simulink model "R7014E_DoubleTankSim2018b_works_on_A"  (R2018a)
settings: Solver=ode5  StartTime=0.0  StopTime=500  FixedStep=0.02  RelTol=1e-3  EnableMultiTasking=on
values from neighbouring files (symbols this model uses):
  A = [a_1*(-1/sqrt(2*g*(h1+EqPoint))) 0 ... (first row only)    [myTank.m]
  B = [6.95/36.2; 0]    [myTank.m]
  C = [0 1]    [myTank.m]
  EqPoint = h_2.signals.values(end)    [myTank.m]
  K = (P*C' + N*0)/[0 1]    [myTank.m]
Description:
  | Double tank process simulation model
  | V1.0
  | 
  | Author: Wolfgang Birk, LTU
settings Model: MinMaxOverflowLogging=ForceOff  Creator=wolfgang  LastModifiedBy=oskwij-4
settings DataIOCC: LimitDataPoints=on  SaveFormat=Array  SignalLoggingSaveFormat=ModelDataLogs
settings OptimizationCC: ExpressionDepthLimit=2147483647  LifeSpan=inf
settings DebuggingCC: UnderspecifiedInitializationDetection=Classic  MergeDetectMultiDrivingBlocksExec=none  SolverPrmCheckMsg=warning  FcnCallInpInsideContextMsg=warning  StateNameClashWarn=warning  SFUnexpectedBacktrackingDiag=warning  SFNoUnconditionalDefaultTransitionDiag=warning  SFExecutionAtInitializationDiag=none
settings HardwareCC: ProdBitPerPointer=32  ProdBitPerSizeT=32  ProdBitPerPtrDiffT=32  ProdLargestAtomicFloat=None  ProdIntDivRoundTo=Undefined  ProdEndianess=Unspecified  ProdWordSize=32  ProdHWDeviceType=32-bit Generic
settings ModelReferenceCC: PropagateSignalLabelsOutOfModel=off
settings CodeAppCC: StateflowObjectComments=on
settings GRTTargetCC: TargetLangStandard=C89/C90 (ANSI)  GeneratePreprocessorConditionals=Disable all
settings ConfigComp: CovMetricSettings=dw  CovHtmlReporting=on  CovSaveCumulativeToWorkspaceVar=on  CovSaveSingleToWorkspaceVar=on  CovExternalEMLEnable=off

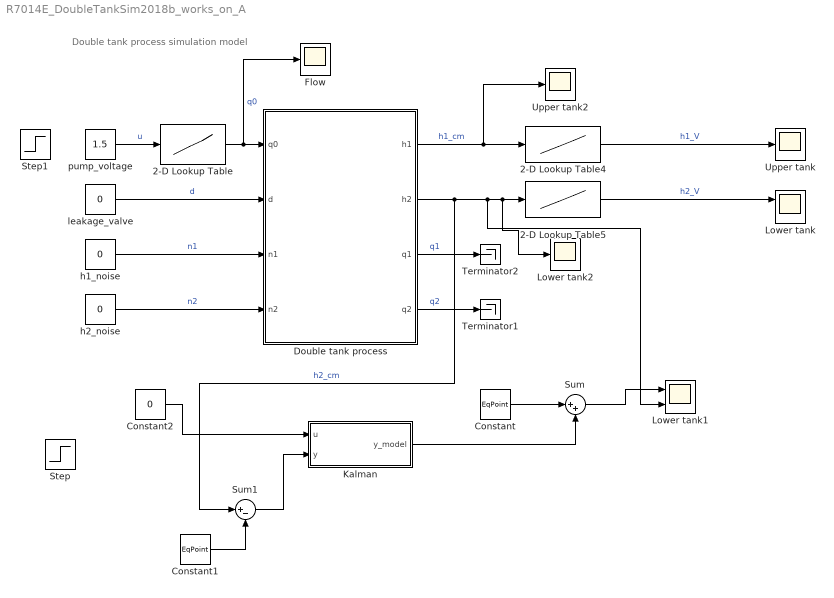
== system R7014E_DoubleTankSim2018b_works_on_A ==
  note: Double tank process simulation model
  2-D Lookup Table : Lookup_n-D  NumberOfTableDimensions=1  BreakpointsForDimension1=x  BreakpointsForDimension2=[1:3]  Table=y  RndMeth=Simplest  InputSameDT=on  mask{x=[0,1,2,3,4,5,6,7,8,9,10], y=[0, 22.23, 28.39, 33.5, 37.5, 41.0, 43.18, 46.9, 48.58, 50.37, 52.97]}
      mask prompts: x "Values on x-axis"; y "Values on y-axis"
  2-D Lookup Table4 : Lookup_n-D  NumberOfTableDimensions=1  BreakpointsForDimension1=x  BreakpointsForDimension2=[1:3]  Table=y  RndMeth=Simplest  InputSameDT=on  mask{x=[0, 2.9, 5.3, 6.5, 8.0, 9.0, 10.1, 11.1, 12.3, 14.0, 15.1], y=[0, 0.47, 2.27, 3.2, 4.3, 5.2, 6.1, 6.8, 7.75, 8.9, 9.8]}
      mask prompts: x "Values on x-axis"; y "Values on y-axis"
  2-D Lookup Table5 : Lookup_n-D  NumberOfTableDimensions=1  BreakpointsForDimension1=x  BreakpointsForDimension2=[1:3]  Table=y  RndMeth=Simplest  InputSameDT=on  mask{x=[0, 3.0, 5.4, 6.9, 7.6, 8.5, 9.5, 10.5, 12.1, 13.6, 14.6], y=[0, 0.83, 2.68, 3.9, 4.5, 5.2, 6.0, 6.9, 8.4, 9.4, 10.0]}
      mask prompts: x "Values on x-axis"; y "Values on y-axis"
  Constant : Constant  Value=EqPoint
  Constant1 : Constant  Value=EqPoint
  Constant2 : Constant  Value=0
  Double tank process : Subsystem  mask{At=33, Ao=0.17, hmax=15.5}
      mask prompts: At "Tank area (cm^2)"; Ao "Opening area (cm^2)"; hmax "Tank height (cm)"
      mask help: Double tank process parameters
  Flow : Scope
  Kalman : Subsystem
  Lower tank : Scope  NumInputPorts=2
  Lower tank1 : Scope  NumInputPorts=2
  "Lower tank2 " : Scope
  Step : Step  Time=250  After=0.1  SampleTime=0
  Step1 : Step  Time=250  Before=2  After=2.1  SampleTime=0
  Sum : Sum  Inputs=|++
  Sum1 : Sum  Inputs=|+-
  Terminator1 : Terminator
  Terminator2 : Terminator
  Upper tank : Scope
  Upper tank2 : Scope
  h1_noise : Constant  Value=0
  h2_noise : Constant  Value=0
  leakage_valve : Constant  Value=0
  pump_voltage : Constant  Value=1.5
  wires:
  2-D Lookup Table4/1 -> Upper tank/1  "h1_V"
  leakage_valve/1 -> Double tank process/2(d)  "d"
  2-D Lookup Table/1 -> Flow/1, Double tank process/1(q0)  "q0"
  Double tank process/1(h1) -> Upper tank2/1, 2-D Lookup Table4/1  "h1_cm"
  Double tank process/2(h2) -> Sum1/1, Lower tank1/2, "Lower tank2 "/1, 2-D Lookup Table5/1  "h2_cm"
  Double tank process/4(q2) -> Terminator1/1  "q2"
  2-D Lookup Table5/1 -> Lower tank/1  "h2_V"
  Double tank process/3(q1) -> Terminator2/1  "q1"
  h1_noise/1 -> Double tank process/3(n1)  "n1"
  h2_noise/1 -> Double tank process/4(n2)  "n2"
  Kalman/1("y_model ") -> Sum/2
  Constant/1 -> Sum/1
  Sum/1 -> Lower tank1/1
  Constant1/1 -> Sum1/2
  Sum1/1 -> Kalman/2(y)
  Constant2/1 -> Kalman/1(u)
  pump_voltage/1 -> 2-D Lookup Table/1  "u"

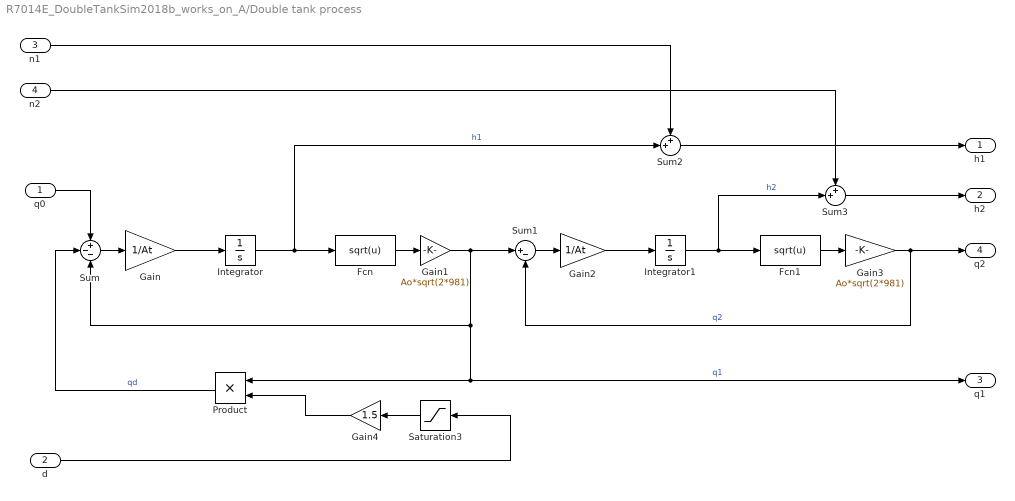
== system R7014E_DoubleTankSim2018b_works_on_A/Double tank process ==
  q0 : Inport
  d : Inport  Port=2
  n1 : Inport  Port=3
  n2 : Inport  Port=4
  Fcn : Fcn  Expr=sqrt(u)
  Fcn1 : Fcn  Expr=sqrt(u)
  Gain : Gain  Gain=1/At
  Gain1 : Gain  Gain=Ao*sqrt(2*981)
  Gain2 : Gain  Gain=1/At
  Gain3 : Gain  Gain=Ao*sqrt(2*981)
  Gain4 : Gain  Gain=1.5
  Integrator : Integrator  InitialCondition=EqPoint  LimitOutput=on  UpperSaturationLimit=hmax  LowerSaturationLimit=0
  Integrator1 : Integrator  InitialCondition=EqPoint  LimitOutput=on  UpperSaturationLimit=hmax  LowerSaturationLimit=0
  Product : Product  RndMeth=Zero
  Saturation3 : Saturate  UpperLimit=1  LowerLimit=0
  Sum : Sum  Inputs=+--
  Sum1 : Sum  Inputs=|+-
  Sum2 : Sum  Inputs=++|
  Sum3 : Sum  Inputs=++|
  h1 : Outport
  h2 : Outport  Port=2
  q1 : Outport  Port=3
  q2 : Outport  Port=4
  wires:
  Sum/1 -> Gain/1
  Gain/1 -> Integrator/1
  Fcn/1 -> Gain1/1
  Gain1/1 -> Sum1/1, Product/1, q1/1, Sum/3  "q1"
  Sum1/1 -> Gain2/1
  Gain2/1 -> Integrator1/1
  Fcn1/1 -> Gain3/1
  Gain3/1 -> Sum1/2, q2/1  "q2"
  q0/1 -> Sum/1
  Integrator/1 -> Sum2/2, Fcn/1  "h1"
  Product/1 -> Sum/2  "qd"
  d/1 -> Saturation3/1
  Integrator1/1 -> Sum3/2, Fcn1/1  "h2"
  Saturation3/1 -> Gain4/1
  Gain4/1 -> Product/2
  Sum2/1 -> h1/1
  n1/1 -> Sum2/1
  Sum3/1 -> h2/1
  n2/1 -> Sum3/1

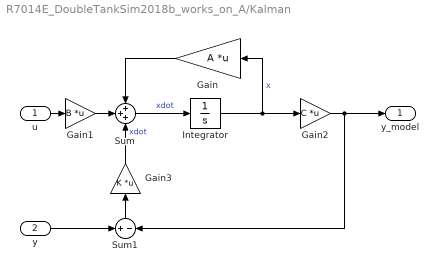
== system R7014E_DoubleTankSim2018b_works_on_A/Kalman ==
  u : Inport
  y : Inport  Port=2
  Gain : Gain  Gain=A  Multiplication=Matrix(K*u)
  Gain1 : Gain  Gain=B  Multiplication=Matrix(K*u)
  Gain2 : Gain  Gain=C  Multiplication=Matrix(K*u)
  Gain3 : Gain  Gain=K  Multiplication=Matrix(K*u)
  Integrator : Integrator
  Sum : Sum  Inputs=+++
  Sum1 : Sum  Inputs=+|-
  "y_model " : Outport
  wires:
  Sum/1 -> Integrator/1  "xdot"
  Integrator/1 -> Gain2/1, Gain/1  "x"
  Gain1/1 -> Sum/2
  u/1 -> Gain1/1
  Gain2/1 -> "y_model "/1, Sum1/2
  y/1 -> Sum1/1
  Sum1/1 -> Gain3/1
  Gain/1 -> Sum/1
  Gain3/1 -> Sum/3  "xdot"
